simulink model "xoxingxitong111"  (Simulink 7.4)
settings: Solver=ode23tb  StartTime=0.0  StopTime=5
undefined symbols (not defined in the file or in its folder): D1, Delta
libraries: powerlib x18
settings Model: Creator=admini  LastModifiedBy=admini
settings DataIOCC: LoadInitialState=on  SaveFinalState=on

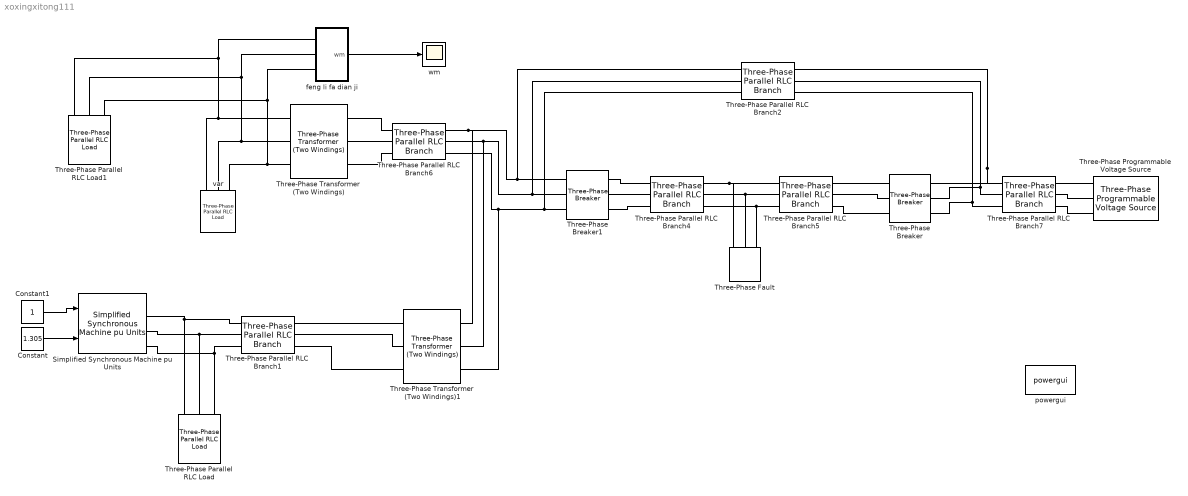
== system xoxingxitong111 ==
  Constant : Constant  Value=1.305  OutDataType=fixdt(1, 16)  OutScaling=2^0
  Constant1 : Constant  OutDataType=fixdt(1, 16)  OutScaling=2^0
  Simplified Synchronous Machine pu Units : powerlib/Machines/Simplified Synchronous Machine pu Units  DialogController=POWERSYS.PowerSysDialog  SystemSampleTime=-1  ConnectionType=3-wire Y  MechanicalLoad=Speed w  NominalParameters=[100e6 13800 50]  Mechanical=[3.7 0 20]  InternalRL="[0.02  0.3]"  InitialConditions="[ 0,0   0,0,0   0,0,0 ]"  Units=0  LoadFlowParameters=[1,0,0,0,0]  TsPowergui=0  TsBlock=-1
  Three-Phase Parallel RLC Branch{1,4,6..7} (4 alike) : powerlib/Elements/Three-Phase Parallel RLC Branch  DialogController=POWERSYS.PowerSysDialog  PhysicalDomain=powersysdomain  SubClassName=unknown  LeftPortType=p1  RightPortType=p1  LConnTagsString=A|B|C  RConnTagsString=A|B|C  BranchType=RLC  Resistance=2  Inductance=0.01  Capacitance=2e-6  Measurements=None
  Three-Phase Parallel RLC Branch2 : powerlib/Elements/Three-Phase Parallel RLC Branch  DialogController=POWERSYS.PowerSysDialog  PhysicalDomain=powersysdomain  SubClassName=unknown  LeftPortType=p1  RightPortType=p1  LConnTagsString=A|B|C  RConnTagsString=A|B|C  BranchType=RLC  Resistance=4  Inductance=0.02  Capacitance=4e-6  Measurements=None
  Three-Phase Parallel RLC Branch5 : powerlib/Elements/Three-Phase Parallel RLC Branch  DialogController=POWERSYS.PowerSysDialog  PhysicalDomain=powersysdomain  SubClassName=unknown  LeftPortType=p1  RightPortType=p1  LConnTagsString=A|B|C  RConnTagsString=A|B|C  BranchType=RLC  Resistance=2  Inductance=0.01  Capacitance=1.0  Measurements=None
  Three-Phase Parallel RLC Load : powerlib/Elements/Three-Phase Parallel RLC Load  DialogController=POWERSYS.PowerSysDialog  PhysicalDomain=powersysdomain  SubClassName=unknown  LeftPortType=p1  RightPortType=p1  LConnTagsString=A|B|C  Configuration=Y (grounded)  NominalVoltage=1000  NominalFrequency=60  ActivePower=500e3  InductivePower=100  CapacitivePower=0  Measurements=None
  Three-Phase Parallel RLC Load1 : powerlib/Elements/Three-Phase Parallel RLC Load  DialogController=POWERSYS.PowerSysDialog  PhysicalDomain=powersysdomain  SubClassName=unknown  LeftPortType=p1  RightPortType=p1  LConnTagsString=A|B|C  Configuration=Y (grounded)  NominalVoltage=1000  NominalFrequency=60  ActivePower=500e3  InductivePower=100  CapacitivePower=0  Measurements=None
  Three-Phase Programmable Voltage Source : powerlib/Electrical Sources/Three-Phase Programmable Voltage Source  DialogController=POWERSYS.PowerSysDialog  SystemSampleTime=-1  PositiveSequence="[46669.0476  0 50]"  VariationEntity=None  VariationType=Step  VariationStep=0.5  VariationRate=10  VariationMagnitude=0.3  VariationFrequency=2  VariationTiming=[1 2]  VariationPhaseA=off  Amplitudes=[1 0.8 1.2 1.0]  TimeValues=[0 0.1 0.15 0.2]  HarmonicGeneration=off  HarmonicA=[3 0.2 -25 0]  HarmonicB=[2 0.15 35 2]  Timing="[0.05  3]"
  Three-Phase Transformer (Two Windings) : powerlib/Elements/Three-Phase Transformer (Two Windings)  DialogController=POWERSYS.PowerSysDialog  SystemSampleTime=-1  Winding1Connection=Delta (D1)  UNITS=pu  NominalPower=[ 250e6 , 50 ]  Winding1=[ 690 , 0.002 , 0.08 ]  Winding2Connection=Yg  Winding2=[ 66000 , 0.002 , 0.08 ]  SetSaturation=off  Rm=500  Lm=500  Saturation=[ 0,0 ; 0.0024,1.2 ; 1.0,1.52 ]  Hysteresis=off  DataFile='hysteresis'  SetInitialFlux=off  InitialFluxes=[ 0.8 , -0.8 , 0.7 ]  Measurements=None  MoreParameters=off  BreakLoop=off  DataType=off  TransfoNumber=1
  Three-Phase Transformer (Two Windings)1 : powerlib/Elements/Three-Phase Transformer (Two Windings)  DialogController=POWERSYS.PowerSysDialog  SystemSampleTime=-1  Winding1Connection=Delta (D1)  UNITS=pu  NominalPower=[ 250e6 , 50 ]  Winding1=[ 13800 , 0.002 , 0.08 ]  Winding2Connection=Yg  Winding2=[ 38150 , 0.002 , 0.08 ]  SetSaturation=off  Rm=500  Lm=500  Saturation=[ 0,0 ; 0.0024,1.2 ; 1.0,1.52 ]  Hysteresis=off  DataFile='hysteresis'  SetInitialFlux=off  InitialFluxes=[ 0.8 , -0.8 , 0.7 ]  Measurements=None  MoreParameters=off  BreakLoop=off  DataType=off  TransfoNumber=1
  Three-Phase Breaker : powerlib/Elements/Three-Phase Breaker  DialogController=POWERSYS.PowerSysDialog  SystemSampleTime=-1  InitialState=closed  SwitchA=off  SwitchB=off  SwitchC=off  SwitchTimes="[0.2  1]"  External=off  BreakerResistance=0.001  SnubberResistance=1e6  SnubberCapacitance=inf  Measurements=None
  Three-Phase Breaker1 : powerlib/Elements/Three-Phase Breaker  DialogController=POWERSYS.PowerSysDialog  SystemSampleTime=-1  InitialState=closed  SwitchA=off  SwitchB=off  SwitchC=off  SwitchTimes="[0.2  1]"  External=off  BreakerResistance=0.001  SnubberResistance=1e6  SnubberCapacitance=inf  Measurements=None
  Three-Phase Fault : powerlib/Elements/Three-Phase Fault  DialogController=POWERSYS.PowerSysDialog  SystemSampleTime=-1  FaultA=off  FaultB=off  FaultC=off  FaultResistance=0.001  GroundFault=off  GroundResistance=0.001  External=off  SwitchStatus=[1 0]  SwitchTimes=[0.01 1]  InitialStates=[0 0 1]  SnubberResistance=1e6  SnubberCapacitance=inf  Measurements=None
  feng li fa dian ji : Subsystem
  powergui : powerlib/powergui  Priority=1  SystemSampleTime=-1  SimulationMode=Continuous  SampleTime=50e-6  frequency=50  SPID=off  DisableSnubberDevices=off  DisableRonSwitches=off  DisableVfSwitches=off  SwTol=0  Interpol=off  frequencyindice=50  echomessages=off  HookPort=off  DisplayEquations=off  FunctionMessages=off  EnableUseOfTLC=off  x0status=blocks  RestoreLinks=warning  Frange=[0:2:500]  Ylog=off  Xlog=on  ShowGrid=off  save=off  variable=ZData  ZoomFFT=on  StartTime=0.0  cycles=1  DisplayStyle=1  fundamental=60  FreqAxis=off  MaxFrequency=1000  frequencyindicesteady=1  RmsSteady=1  display=off  Ts=0  methode=off
  var : powerlib/Elements/Three-Phase Parallel RLC Load  DialogController=POWERSYS.PowerSysDialog  PhysicalDomain=powersysdomain  SubClassName=unknown  LeftPortType=p1  RightPortType=p1  LConnTagsString=A|B|C  Configuration=Delta  NominalVoltage=690  NominalFrequency=50  ActivePower=0  InductivePower=0  CapacitivePower=10000e3  Measurements=None
  wm : Scope
      settings: TimeRange=5  YMin=1.01399  YMax=1.01399  SaveName=lpy  DataFormat=Array
  wires:
  Constant1/1 -> Simplified Synchronous Machine pu Units/1
  Constant/1 -> Simplified Synchronous Machine pu Units/2
  feng li fa dian ji/1(wm) -> wm/1
  connections:
  Simplified Synchronous Machine pu Units/RConn3 -- Three-Phase Parallel RLC Branch1/LConn3 -- Three-Phase Parallel RLC Load/LConn3
  Simplified Synchronous Machine pu Units/RConn2 -- Three-Phase Parallel RLC Branch1/LConn2 -- Three-Phase Parallel RLC Load/LConn2
  Three-Phase Parallel RLC Load/LConn1 -- Three-Phase Parallel RLC Branch1/LConn1 -- Simplified Synchronous Machine pu Units/RConn1
  Three-Phase Parallel RLC Branch1/RConn2 -- Three-Phase Transformer (Two Windings)1/LConn2
  Three-Phase Parallel RLC Branch1/RConn1 -- Three-Phase Transformer (Two Windings)1/LConn1
  Three-Phase Parallel RLC Branch1/RConn3 -- Three-Phase Transformer (Two Windings)1/LConn3
  Three-Phase Transformer (Two Windings)/LConn1 -- feng li fa dian ji/LConn1 -- Three-Phase Parallel RLC Load1/LConn1 -- var/LConn1
  Three-Phase Parallel RLC Load1/LConn2 -- feng li fa dian ji/LConn2 -- Three-Phase Transformer (Two Windings)/LConn2 -- var/LConn2
  Three-Phase Parallel RLC Load1/LConn3 -- feng li fa dian ji/LConn3 -- var/LConn3 -- Three-Phase Transformer (Two Windings)/LConn3
  Three-Phase Transformer (Two Windings)/RConn1 -- Three-Phase Parallel RLC Branch6/LConn1
  Three-Phase Transformer (Two Windings)/RConn2 -- Three-Phase Parallel RLC Branch6/LConn2
  Three-Phase Transformer (Two Windings)/RConn3 -- Three-Phase Parallel RLC Branch6/LConn3
  Three-Phase Parallel RLC Branch7/RConn3 -- Three-Phase Programmable Voltage Source/RConn3
  Three-Phase Parallel RLC Branch7/RConn1 -- Three-Phase Programmable Voltage Source/RConn1
  Three-Phase Parallel RLC Branch7/RConn2 -- Three-Phase Programmable Voltage Source/RConn2
  Three-Phase Parallel RLC Branch2/RConn2 -- Three-Phase Breaker/RConn2 -- Three-Phase Parallel RLC Branch7/LConn2
  Three-Phase Parallel RLC Branch2/RConn3 -- Three-Phase Parallel RLC Branch7/LConn3 -- Three-Phase Breaker/RConn3
  Three-Phase Parallel RLC Branch2/RConn1 -- Three-Phase Breaker/RConn1 -- Three-Phase Parallel RLC Branch7/LConn1
  Three-Phase Parallel RLC Branch4/LConn1 -- Three-Phase Breaker1/RConn1
  Three-Phase Parallel RLC Branch4/LConn2 -- Three-Phase Breaker1/RConn2
  Three-Phase Parallel RLC Branch4/LConn3 -- Three-Phase Breaker1/RConn3
  Three-Phase Parallel RLC Branch5/RConn1 -- Three-Phase Breaker/LConn1
  Three-Phase Parallel RLC Branch5/RConn2 -- Three-Phase Breaker/LConn2
  Three-Phase Parallel RLC Branch5/RConn3 -- Three-Phase Breaker/LConn3
  Three-Phase Parallel RLC Branch6/RConn1 -- Three-Phase Transformer (Two Windings)1/RConn1 -- Three-Phase Breaker1/LConn1 -- Three-Phase Parallel RLC Branch2/LConn1
  Three-Phase Breaker1/LConn2 -- Three-Phase Parallel RLC Branch6/RConn2 -- Three-Phase Transformer (Two Windings)1/RConn2 -- Three-Phase Parallel RLC Branch2/LConn2
  Three-Phase Parallel RLC Branch6/RConn3 -- Three-Phase Transformer (Two Windings)1/RConn3 -- Three-Phase Breaker1/LConn3 -- Three-Phase Parallel RLC Branch2/LConn3
  Three-Phase Parallel RLC Branch4/RConn1 -- Three-Phase Parallel RLC Branch5/LConn1 -- Three-Phase Fault/LConn1
  Three-Phase Parallel RLC Branch4/RConn2 -- Three-Phase Parallel RLC Branch5/LConn2 -- Three-Phase Fault/LConn2
  Three-Phase Parallel RLC Branch4/RConn3 -- Three-Phase Parallel RLC Branch5/LConn3 -- Three-Phase Fault/LConn3

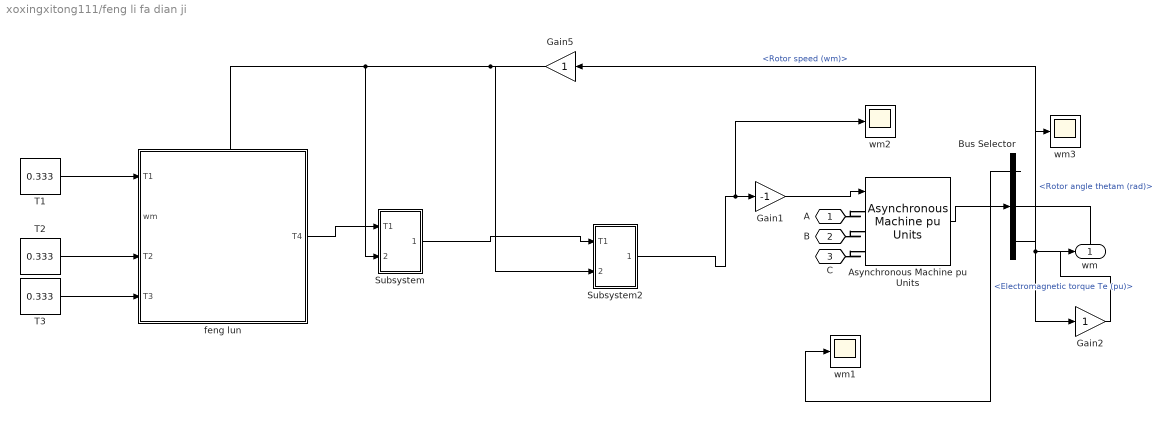
== system xoxingxitong111/feng li fa dian ji ==
  Asynchronous Machine pu Units : powerlib/Machines/Asynchronous Machine pu Units  DialogController=POWERSYS.PowerSysDialog  SystemSampleTime=-1  PresetModel=No  MechanicalLoad=Torque Tm  ShowDetailedParameters=on  RotorType=Squirrel-cage  ReferenceFrame=Rotor  NominalParameters=[50000000 690 50]  Stator=[0.01379 0.04775]  Rotor=[0.007728 0.04775]  Lm=2.416  Mechanical=[0.2838 0.008726 2]  PolePairs=2  InitialConditions="[ -0.1,0   1,1,1  0,0,0 ]"  Units=pu  LoadFlowParameters=0  SimulateSaturation=off  Saturation="[0.212,0.4201,0.8125,1.0979,1.4799,2.2457,3.2586,4.5763,6.4763 ;   0.5,0.7,0.9,1,1.1,1.2 ,1.3,1.4,1.5]"  TsPowergui=0  TsBlock=-1  IterativeModel=Forward Euler
      link override Electrical model/Continuous/Stator/phiqs: InitialCondition=0.00001
      link override Mechanical model/Continuous Tm input/Rotor angle thetam: InitialCondition=0.0001
      link override Mechanical model/Continuous Tm input/Rotor speed (wm): InitialCondition=0.0001
  Bus Selector : BusSelector  OutputSignals=Mechanical.Electromagnetic torque Te (pu),Mechanical.Rotor speed (wm),Mechanical.Rotor angle thetam (rad)
  Gain1 : Gain  Gain=-1  ParameterDataType=fixdt(1, 16)  ParameterScaling=2^0  OutDataType=fixdt(1, 16)  OutScaling=2^0
  Gain2 : Gain  ParameterDataType=fixdt(1, 16)  ParameterScaling=2^0  OutDataType=fixdt(1, 16)  OutScaling=2^0
  Gain5 : Gain  ParameterDataType=fixdt(1, 16)  ParameterScaling=2^0  OutDataType=fixdt(1, 16)  OutScaling=2^0
  Subsystem : Subsystem
  Subsystem2 : Subsystem
  T1 : Constant  Value=0.333  OutDataType=fixdt(1, 16)  OutScaling=2^0
  T2 : Constant  Value=0.333  OutDataType=fixdt(1, 16)  OutScaling=2^0
  T3 : Constant  Value=0.333  OutDataType=fixdt(1, 16)  OutScaling=2^0
  feng lun : Subsystem
  wm1 : Scope
      settings: TimeRange=10  YMin=-0.9625  YMax=-0.9275  SaveName=lpy1  DataFormat=Array
  wm2 : Scope
      settings: TimeRange=5  YMin=0.95225  YMax=0.95725  SaveName=lpy2  DataFormat=Array
  wm3 : Scope
      settings: TimeRange=10  YMin=-1.5  YMax=2  SaveName=lpy5  DataFormat=Array
  A : PMIOPort  Port=1  Side=Left
  B : PMIOPort  Port=2  Side=Left
  C : PMIOPort  Port=3  Side=Left
  wm : Outport
  wires:
  Asynchronous Machine pu Units/1 -> Bus Selector/1
  Bus Selector/2 -> Gain5/1, Gain2/1  "<Rotor speed (wm)>"
  T2/1 -> feng lun/3(T2)
  T3/1 -> feng lun/4(T3)
  T1/1 -> feng lun/1(T1)
  Subsystem2/1(Out1) -> Gain1/1, wm2/1
  Bus Selector/1 -> wm1/1  "<Electromagnetic torque Te (pu)>"
  Gain5/1 -> feng lun/2(wm), Subsystem/2(In2), Subsystem2/2(In2)
  Subsystem/1(Out1) -> Subsystem2/1(T1)
  Gain1/1 -> Asynchronous Machine pu Units/1
  feng lun/1(T4) -> Subsystem/1(T1)
  Gain2/1 -> wm/1
  Bus Selector/3 -> wm3/1  "<Rotor angle thetam (rad)>"
  connections:
  A/RConn1 -- Asynchronous Machine pu Units/LConn1
  B/RConn1 -- Asynchronous Machine pu Units/LConn2
  C/RConn1 -- Asynchronous Machine pu Units/LConn3

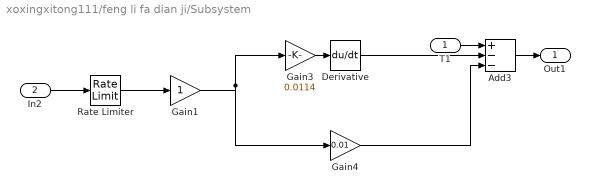
== system xoxingxitong111/feng li fa dian ji/Subsystem ==
  T1 : Inport
  In2 : Inport  Port=2
  Add3 : Sum  Inputs=+--  OutDataType=fixdt(1, 16)  OutScaling=2^-10
  Derivative : Derivative
  Gain1 : Gain  ParameterDataType=fixdt(1, 16)  ParameterScaling=2^0  OutDataType=fixdt(1, 16)  OutScaling=2^0
  Gain3 : Gain  Gain=0.0114  ParameterDataType=fixdt(1, 16)  ParameterScaling=2^0  OutDataType=fixdt(1, 16)  OutScaling=2^0
  Gain4 : Gain  Gain=0.01  ParameterDataType=fixdt(1, 16)  ParameterScaling=2^0  OutDataType=fixdt(1, 16)  OutScaling=2^0
  Rate Limiter : RateLimiter  RisingSlewLimit=100  FallingSlewLimit=-100  SampleTimeMode=inherited  LinearizeAsGain=off
  Out1 : Outport
  wires:
  Gain3/1 -> Derivative/1
  Derivative/1 -> Add3/2
  T1/1 -> Add3/1
  Gain1/1 -> Gain3/1, Gain4/1
  Add3/1 -> Out1/1
  In2/1 -> Rate Limiter/1
  Rate Limiter/1 -> Gain1/1
  Gain4/1 -> Add3/3

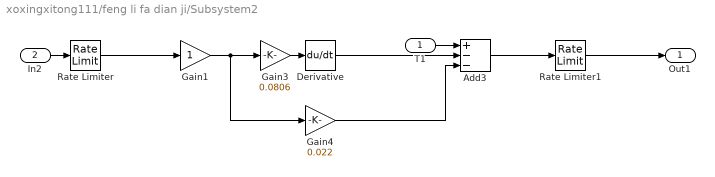
== system xoxingxitong111/feng li fa dian ji/Subsystem2 ==
  T1 : Inport
  In2 : Inport  Port=2
  Add3 : Sum  Inputs=+--  OutDataType=fixdt(1, 16)  OutScaling=2^-10
  Derivative : Derivative
  Gain1 : Gain  ParameterDataType=fixdt(1, 16)  ParameterScaling=2^0  OutDataType=fixdt(1, 16)  OutScaling=2^0
  Gain3 : Gain  Gain=0.0806  ParameterDataType=fixdt(1, 16)  ParameterScaling=2^0  OutDataType=fixdt(1, 16)  OutScaling=2^0
  Gain4 : Gain  Gain=0.022  ParameterDataType=fixdt(1, 16)  ParameterScaling=2^0  OutDataType=fixdt(1, 16)  OutScaling=2^0
  Rate Limiter : RateLimiter  RisingSlewLimit=100  FallingSlewLimit=-100  SampleTimeMode=inherited  LinearizeAsGain=off
  Rate Limiter1 : RateLimiter  RisingSlewLimit=100  FallingSlewLimit=-100  SampleTimeMode=inherited  LinearizeAsGain=off
  Out1 : Outport
  wires:
  Gain3/1 -> Derivative/1
  Derivative/1 -> Add3/2
  T1/1 -> Add3/1
  In2/1 -> Rate Limiter/1
  Add3/1 -> Rate Limiter1/1
  Rate Limiter1/1 -> Out1/1
  Gain4/1 -> Add3/3
  Rate Limiter/1 -> Gain1/1
  Gain1/1 -> Gain3/1, Gain4/1

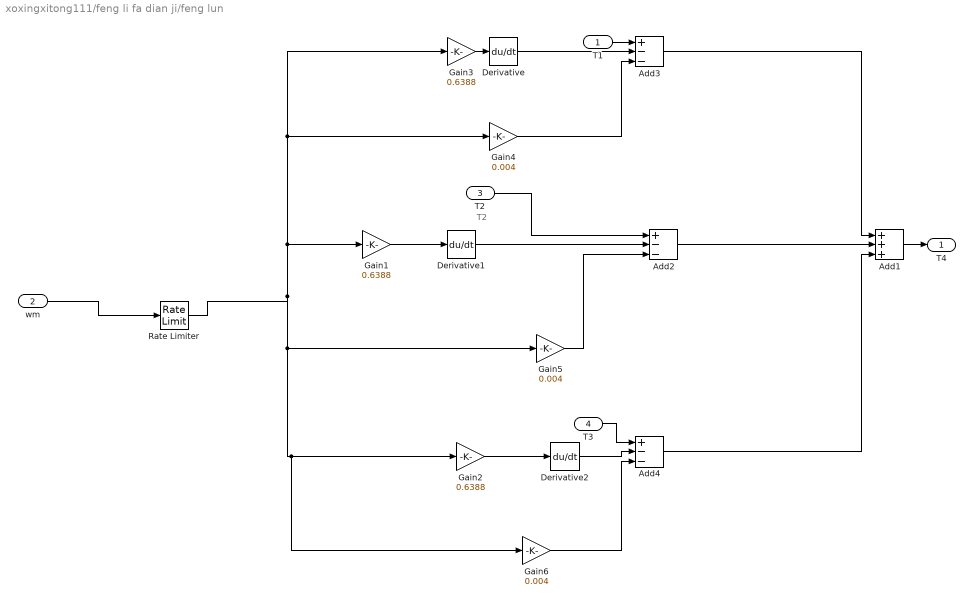
== system xoxingxitong111/feng li fa dian ji/feng lun ==
  note: T2
  T1 : Inport
  wm : Inport  Port=2  OutDataType=fixdt(1, 16)  OutScaling=2^0
  T2 : Inport  Port=3
  T3 : Inport  Port=4
  Add1 : Sum  Inputs=+++  OutDataType=fixdt(1, 16)  OutScaling=2^-10
  Add2 : Sum  Inputs=+--  OutDataType=fixdt(1, 16)  OutScaling=2^-10
  Add3 : Sum  Inputs=+--  OutDataType=fixdt(1, 16)  OutScaling=2^-10
  Add4 : Sum  Inputs=+--  OutDataType=fixdt(1, 16)  OutScaling=2^-10
  Derivative : Derivative
  Derivative1 : Derivative
  Derivative2 : Derivative
  Gain1 : Gain  Gain=0.6388  ParameterDataType=fixdt(1, 16)  ParameterScaling=2^0  OutDataType=fixdt(1, 16)  OutScaling=2^0
  Gain2 : Gain  Gain=0.6388  ParameterDataType=fixdt(1, 16)  ParameterScaling=2^0  OutDataType=fixdt(1, 16)  OutScaling=2^0
  Gain3 : Gain  Gain=0.6388  ParameterDataType=fixdt(1, 16)  ParameterScaling=2^0  OutDataType=fixdt(1, 16)  OutScaling=2^0
  Gain4 : Gain  Gain=0.004  ParameterDataType=fixdt(1, 16)  ParameterScaling=2^0  OutDataType=fixdt(1, 16)  OutScaling=2^0
  Gain5 : Gain  Gain=0.004  ParameterDataType=fixdt(1, 16)  ParameterScaling=2^0  OutDataType=fixdt(1, 16)  OutScaling=2^0
  Gain6 : Gain  Gain=0.004  ParameterDataType=fixdt(1, 16)  ParameterScaling=2^0  OutDataType=fixdt(1, 16)  OutScaling=2^0
  Rate Limiter : RateLimiter  RisingSlewLimit=100  FallingSlewLimit=-100  SampleTimeMode=inherited  LinearizeAsGain=off
  T4 : Outport
  wires:
  Add3/1 -> Add1/1
  Add4/1 -> Add1/3
  Gain3/1 -> Derivative/1
  Derivative/1 -> Add3/2
  Gain1/1 -> Derivative1/1
  Gain2/1 -> Derivative2/1
  Derivative2/1 -> Add4/2
  Add2/1 -> Add1/2
  Gain4/1 -> Add3/3
  Gain6/1 -> Add4/3
  Add1/1 -> T4/1
  T1/1 -> Add3/1
  T3/1 -> Add4/1
  T2/1 -> Add2/1
  Derivative1/1 -> Add2/2
  Gain5/1 -> Add2/3
  wm/1 -> Rate Limiter/1
  Rate Limiter/1 -> Gain1/1, Gain3/1, Gain4/1, Gain2/1, Gain6/1, Gain5/1
